simulink model "P1"  (R2019b)
settings: Solver=VariableStepAuto  StartTime=0.0  StopTime=20  RelTol=1e-3
values from neighbouring files (symbols this model uses):
  x1_0 = 2.*rand(1,1)-1    [p1_initialization.m]    (also in p3_initialization.m; p4_initialization.m = 1)
  x2_0 = 2.*rand(1,1)-1    [p1_initialization.m]    (also in p3_initialization.m; p4_initialization.m = -1)
  x3_0 = 2.*rand(1,1)-1    [p1_initialization.m]    (also in p3_initialization.m; p4_initialization.m = 3)
  x4_0 = 2.*rand(1,1)-1    [p1_initialization.m]    (also in p3_initialization.m; p4_initialization.m = 1)
  x5_0 = 2.*rand(1,1)-1    [p1_initialization.m]
settings Model: Creator=cz  LastModifiedBy=cz

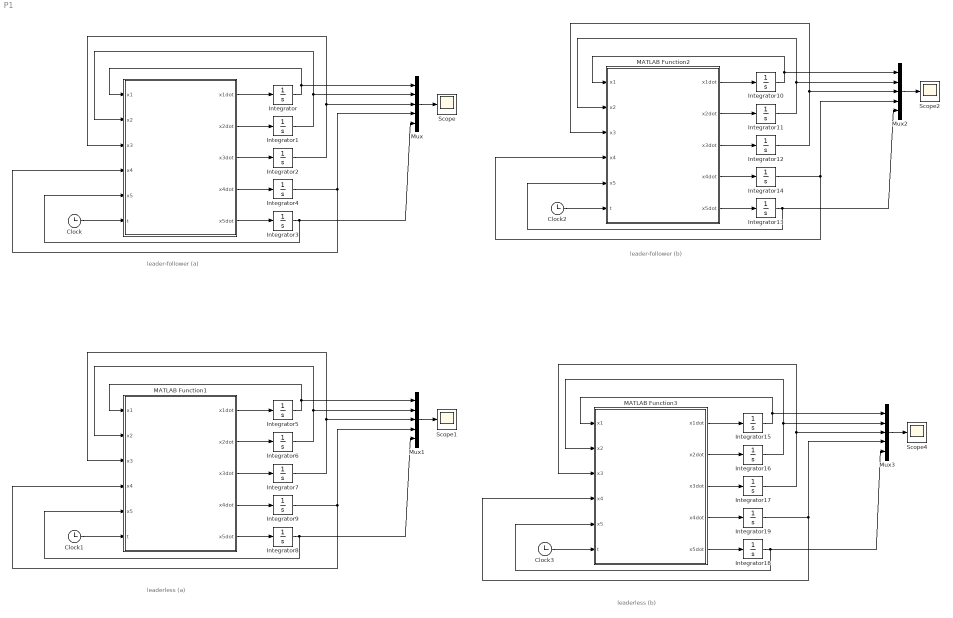
== system P1 ==
  note: leader-follower (b)
  note: leader-follower (a)
  note: leaderless (a)
  note: leaderless (b)
  " " : MATLAB Function  TreatAsAtomicUnit=on
  Clock{,1..3} (4 alike) : Clock
  Integrator{,5,10,15} (4 alike) : Integrator  InitialCondition=x1_0
  Integrator{1,6,11,16} (4 alike) : Integrator  InitialCondition=x2_0
  Integrator{2,7,12,17} (4 alike) : Integrator  InitialCondition=x3_0
  Integrator{3,8,13,18} (4 alike) : Integrator  InitialCondition=x5_0
  Integrator{4,9,14,19} (4 alike) : Integrator  InitialCondition=x4_0
  MATLAB Function1 : MATLAB Function  TreatAsAtomicUnit=on
  MATLAB Function2 : MATLAB Function  TreatAsAtomicUnit=on
  MATLAB Function3 : MATLAB Function  TreatAsAtomicUnit=on
  Mux{,1..3} (4 alike) : Mux  Inputs=5
  Scope{,1..2,4} (4 alike) : Scope
  wires:
  " "/5(x5dot) -> Integrator3/1
  " "/1(x1dot) -> Integrator/1
  " "/2(x2dot) -> Integrator1/1
  " "/3(x3dot) -> Integrator2/1
  " "/4(x4dot) -> Integrator4/1
  Integrator/1 -> Mux/1, " "/1(x1)
  Integrator1/1 -> Mux/2, " "/2(x2)
  Integrator2/1 -> Mux/3, " "/3(x3)
  Integrator4/1 -> " "/4(x4), Mux/4
  Integrator3/1 -> " "/5(x5), Mux/5
  Mux/1 -> Scope/1
  Clock/1 -> " "/6(t)
  Mux1/1 -> Scope1/1
  Clock1/1 -> MATLAB Function1/6(t)
  Integrator6/1 -> Mux1/2, MATLAB Function1/2(x2)
  Integrator8/1 -> MATLAB Function1/5(x5), Mux1/5
  MATLAB Function1/5(x5dot) -> Integrator8/1
  Integrator7/1 -> Mux1/3, MATLAB Function1/3(x3)
  Integrator5/1 -> Mux1/1, MATLAB Function1/1(x1)
  MATLAB Function1/3(x3dot) -> Integrator7/1
  MATLAB Function1/4(x4dot) -> Integrator9/1
  Integrator9/1 -> MATLAB Function1/4(x4), Mux1/4
  MATLAB Function1/1(x1dot) -> Integrator5/1
  MATLAB Function1/2(x2dot) -> Integrator6/1
  Mux2/1 -> Scope2/1
  Integrator11/1 -> Mux2/2, MATLAB Function2/2(x2)
  Integrator13/1 -> MATLAB Function2/5(x5), Mux2/5
  MATLAB Function2/5(x5dot) -> Integrator13/1
  Integrator12/1 -> Mux2/3, MATLAB Function2/3(x3)
  Integrator10/1 -> Mux2/1, MATLAB Function2/1(x1)
  MATLAB Function2/3(x3dot) -> Integrator12/1
  MATLAB Function2/4(x4dot) -> Integrator14/1
  Integrator14/1 -> MATLAB Function2/4(x4), Mux2/4
  MATLAB Function2/1(x1dot) -> Integrator10/1
  MATLAB Function2/2(x2dot) -> Integrator11/1
  Clock2/1 -> MATLAB Function2/6(t)
  Integrator18/1 -> MATLAB Function3/5(x5), Mux3/5
  Integrator16/1 -> Mux3/2, MATLAB Function3/2(x2)
  Mux3/1 -> Scope4/1
  MATLAB Function3/2(x2dot) -> Integrator16/1
  Integrator19/1 -> MATLAB Function3/4(x4), Mux3/4
  Clock3/1 -> MATLAB Function3/6(t)
  MATLAB Function3/4(x4dot) -> Integrator19/1
  MATLAB Function3/5(x5dot) -> Integrator18/1
  MATLAB Function3/3(x3dot) -> Integrator17/1
  MATLAB Function3/1(x1dot) -> Integrator15/1
  Integrator15/1 -> Mux3/1, MATLAB Function3/1(x1)
  Integrator17/1 -> Mux3/3, MATLAB Function3/3(x3)

== matlab function P1/MATLAB Function1 ==
  data: x1 input; x1dot output; x2 input; x3 input; x4 input; x5 input; x2dot output; x3dot output; x4dot output; x5dot output; t input
function [x1dot,x2dot,x3dot,x4dot,x5dot] = fcn(x1,x2,x3,x4,x5,t)
x1dot=x5-x1;
x2dot=x1-x2;
x3dot=x2-x3;
x4dot=x3-x4;
x5dot=x4-x5;

== matlab function P1/  ==
  data: x1 input; x1dot output; x2 input; x3 input; x4 input; x5 input; x2dot output; x3dot output; x4dot output; x5dot output; t input
function [x1dot,x2dot,x3dot,x4dot,x5dot] = fcn(x1,x2,x3,x4,x5,t)
k=10;
x1dot=0;
x2dot=k*(x1-x2);
x3dot=k*(x2-x3);
x4dot=k*(x3-x4);
x5dot=k*(x1-x5);

== matlab function P1/MATLAB Function2 ==
  data: x1 input; x1dot output; x2 input; x3 input; x4 input; x5 input; x2dot output; x3dot output; x4dot output; x5dot output; t input
function [x1dot,x2dot,x3dot,x4dot,x5dot] = fcn(x1,x2,x3,x4,x5,t)
k=10;
x1dot=0;
if t>1
    x2dot=0;
else
    x2dot=k*(x1-x2);
end
x3dot=k*(x2-x3);
x4dot=k*(x3-x4);
x5dot=k*(x1-x5);

== matlab function P1/MATLAB Function3 ==
  data: x1 input; x1dot output; x2 input; x3 input; x4 input; x5 input; x2dot output; x3dot output; x4dot output; x5dot output; t input
function [x1dot,x2dot,x3dot,x4dot,x5dot] = fcn(x1,x2,x3,x4,x5,t)
x1dot=x5-x1;
if t>1
    x2dot=0;
else
    x2dot=x1-x2;
end
x3dot=x2-x3;
x4dot=x3-x4;
x5dot=x4-x5;
